simulink model "Three_torques_inputs"  (R2015a)
settings: Solver=ode45  SolverMode=SingleTasking  StartTime=0.0  StopTime=10.0  MaxStep=0.01  RelTol=1e-3
values from neighbouring files (symbols this model uses):
  A = eval(As)    [Three_torque_input.m]    (also in fourinputslq_and_yaw_rate_control.m; linearization.m)
  B = eval(Bs)    [Three_torque_input.m]    (also in fourinputslq_and_yaw_rate_control.m; linearization.m)
  Cs = [1 0 0 0 0 0; 0 1 0 0 0 0; 0 0 1 0 0 0;  0 0 0 1 0 0;0 0 0 0 1 0]    [Three_torque_input.m]    (also in fourinputslq_and_yaw_rate_control.m; linearization.m)
  Kr = -inv(Cc*inv(Aa-Bb*K)*Bb)    [Three_torque_input.m]    (also in fourinputslq_and_yaw_rate_control.m = -inv(Cc*inv(Aa-Bb*K)*Bb(:,2:4)); linearization.m = -inv(Cc*inv(Aa-Bb*Kk-eye(5))*Bb))
undefined symbols (not defined in the file or in its folder): K
settings Model: Creator=Jaby  LastModifiedBy=Jaby
settings OptimizationCC: BlockReduction=off  BooleanDataType=off
settings DebuggingCC: SaveWithParameterizedLinksMsg=none  UnderspecifiedInitializationDetection=Classic  MergeDetectMultiDrivingBlocksExec=none  SignalResolutionControl=TryResolveAllWithWarning
settings HardwareCC: TargetUnknown=on

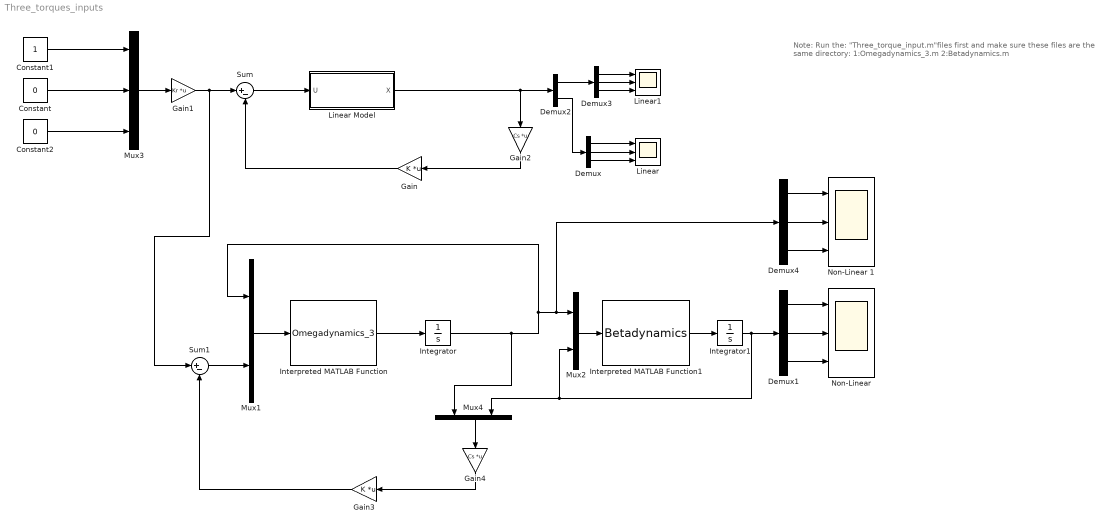
== system Three_torques_inputs ==
  note: Note:
      | Run the: "Three_torque_input.m"files first
      | and make sure these files are the same directory:
      | 1:Omegadynamics_3.m
      | 2:Betadynamics.m
  Constant : Constant  Value=0  VectorParams1D=off
  Constant1 : Constant  VectorParams1D=off
  Constant2 : Constant  Value=0  VectorParams1D=off
  Demux{,1,3..4} (4 alike) : Demux  Outputs=3
  Demux2 : Demux  Outputs=2
  Gain : Gain  Gain=K  Multiplication=Matrix(K*u)
  Gain1 : Gain  Gain=Kr  Multiplication=Matrix(K*u)
  Gain2 : Gain  Gain=Cs  Multiplication=Matrix(K*u)
  Gain3 : Gain  Gain=K  Multiplication=Matrix(K*u)
  Gain4 : Gain  Gain=Cs  Multiplication=Matrix(K*u)
  Integrator : Integrator  InitialCondition=[0 0 0]'
  Integrator1 : Integrator  InitialCondition=[0 0 0]'
  Interpreted MATLAB Function : MATLABFcn  MATLABFcn=Omegadynamics_3  Output1D=off
  Interpreted MATLAB Function1 : MATLABFcn  MATLABFcn=Betadynamics  Output1D=off
  Linear : Scope  NumInputPorts=3
      settings: TimeRange=20  YMin=0.00274~-3.07e-14~8.3e-31  YMax=0.00278~-3.025e-14~8.43e-31
  "Linear Model " : Subsystem
  Linear1 : Scope  NumInputPorts=3
      settings: TimeRange=20  YMin=-0.5~-0.5~0  YMax=2.5~2.5~0.7000000000000001  SaveName=ScopeData2
  Mux1 : Mux  Inputs=2
  Mux2 : Mux  Inputs=2
  Mux3 : Mux  Inputs=3
  Mux4 : Mux  Inputs=2
  "Non-Linear " : Scope  NumInputPorts=3
      settings: YMin=-5~-5~-5  YMax=5~5~5
  Non-Linear 1 : Scope  NumInputPorts=3
      settings: TimeRange=10  YMin=-5~-5~-5  YMax=5~5~5  SaveName=ScopeData3
  Sum : Sum  Inputs=|+-
  Sum1 : Sum  Inputs=|+-
  wires:
  "Linear Model "/1(X) -> Demux2/1, Gain2/1
  Demux/1 -> Linear/1
  Demux/2 -> Linear/2
  Demux/3 -> Linear/3
  Mux1/1 -> Interpreted MATLAB Function/1
  Interpreted MATLAB Function/1 -> Integrator/1
  Interpreted MATLAB Function1/1 -> Integrator1/1
  Demux1/2 -> "Non-Linear "/2
  Integrator1/1 -> Demux1/1, Mux4/2, Mux2/2
  Demux1/3 -> "Non-Linear "/3
  Demux1/1 -> "Non-Linear "/1
  Mux2/1 -> Interpreted MATLAB Function1/1
  Sum/1 -> "Linear Model "/1(U)
  Gain/1 -> Sum/2
  Demux2/2 -> Demux/1
  Mux3/1 -> Gain1/1
  Gain1/1 -> Sum1/1, Sum/1
  Constant/1 -> Mux3/2
  Constant1/1 -> Mux3/1
  Demux3/1 -> Linear1/1
  Demux3/2 -> Linear1/2
  Demux3/3 -> Linear1/3
  Demux2/1 -> Demux3/1
  Constant2/1 -> Mux3/3
  Gain2/1 -> Gain/1
  Gain3/1 -> Sum1/2
  Gain4/1 -> Gain3/1
  Mux4/1 -> Gain4/1
  Sum1/1 -> Mux1/2
  Demux4/2 -> Non-Linear 1/2
  Integrator/1 -> Mux4/1, Demux4/1, Mux2/1, Mux1/1
  Demux4/3 -> Non-Linear 1/3
  Demux4/1 -> Non-Linear 1/1

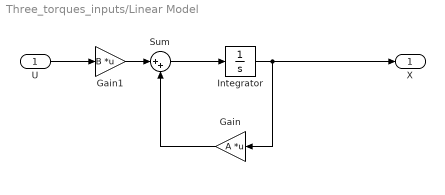
== system Three_torques_inputs/Linear Model  ==
  U : Inport
  Gain : Gain  Gain=A  Multiplication=Matrix(K*u)
  Gain1 : Gain  Gain=B  Multiplication=Matrix(K*u)
  Integrator : Integrator
  Sum : Sum  Inputs=|++
  X : Outport
  wires:
  Integrator/1 -> X/1, Gain/1
  U/1 -> Gain1/1
  Gain1/1 -> Sum/1
  Sum/1 -> Integrator/1
  Gain/1 -> Sum/2
